simulink model "NCMS_AltMis_항공대"  (R2022a)
settings: Solver=FixedStepAuto  StartTime=0.0  StopTime=inf  FixedStep=SampleTime  RelTol=1e-3
InitFcn:
  | NCMS_AltMis_Init;
values from neighbouring files (symbols this model uses):
  Kdpr = 0.004    [NCMS_AltMis_Init_항공대.m]
  Kdrr = 0.004    [NCMS_AltMis_Init_항공대.m]
  Kdvz = 0.0254    [NCMS_AltMis_Init_항공대.m]
  Kdyr = 0.0298    [NCMS_AltMis_Init_항공대.m]
  Kipr = 0.1    [NCMS_AltMis_Init_항공대.m]
  Kirr = 0.1    [NCMS_AltMis_Init_항공대.m]
  Kivx = 0.0728/g    (= 0.00742099898063)    [NCMS_AltMis_Init_항공대.m]
  Kivy = 0.0728/g    (= 0.00742099898063)    [NCMS_AltMis_Init_항공대.m]
  Kivz = 0.6304    [NCMS_AltMis_Init_항공대.m]
  Kix = 0.02    [NCMS_AltMis_Init_항공대.m]
  Kiyaxis = 0.02    [NCMS_AltMis_Init_항공대.m]
  Kiyr = 0.7395    [NCMS_AltMis_Init_항공대.m]
  Kiz = 0.09    [NCMS_AltMis_Init_항공대.m]
  Kpp = 3.3894    [NCMS_AltMis_Init_항공대.m]
  Kppr = 0.1    [NCMS_AltMis_Init_항공대.m]
  Kpr = 3.3894    [NCMS_AltMis_Init_항공대.m]
  Kprr = 0.1    [NCMS_AltMis_Init_항공대.m]
  Kpvx = 2.1109/g    (= 0.215178389399)    [NCMS_AltMis_Init_항공대.m]
  Kpvy = 2.1109/g    (= 0.215178389399)    [NCMS_AltMis_Init_항공대.m]
  Kpvz = 0.3191    [NCMS_AltMis_Init_항공대.m]
  Kpx = 1    [NCMS_AltMis_Init_항공대.m]
  Kpy = 3.3894    [NCMS_AltMis_Init_항공대.m]
  Kpyaxis = 1    [NCMS_AltMis_Init_항공대.m]
  Kpyr = 0.3744    [NCMS_AltMis_Init_항공대.m]
  Kpz = 2.4    [NCMS_AltMis_Init_항공대.m]
  LAND_PRES_VEL = 0.2    [NCMS_AltMis_Init_항공대.m]
  MAX_CONTROL_ANGLE_PITCH = 30*pi/180    (= 0.523598775598)    [Init_FLIGHT_Hexacopter.m]    (also in NCMS_AltMis_Init_항공대.m = 0.349065850399)
  MAX_CONTROL_ANGLE_RATE_PITCH = 360*pi/180    (= 6.28318530718)    [Init_FLIGHT_Hexacopter.m]    (also in NCMS_AltMis_Init_항공대.m)
  MAX_CONTROL_ANGLE_RATE_ROLL = 360*pi/180    (= 6.28318530718)    [Init_FLIGHT_Hexacopter.m]    (also in NCMS_AltMis_Init_항공대.m)
  MAX_CONTROL_ANGLE_RATE_Y = 120*pi/180    (= 2.09439510239)    [Init_FLIGHT_Hexacopter.m]    (also in NCMS_AltMis_Init_항공대.m)
  MAX_CONTROL_ANGLE_ROLL = 30*pi/180    (= 0.523598775598)    [Init_FLIGHT_Hexacopter.m]    (also in NCMS_AltMis_Init_항공대.m = 0.349065850399)
  MAX_CONTROL_VELOCITY_XY = 1.5    [Init_FLIGHT_Hexacopter.m]    (also in NCMS_AltMis_Init_항공대.m)
  MAX_CONTROL_VELOCITY_Z = 1    [Init_FLIGHT_Hexacopter.m]    (also in NCMS_AltMis_Init_항공대.m)
  Npr = 50    [NCMS_AltMis_Init_항공대.m]
  Nrr = 50    [NCMS_AltMis_Init_항공대.m]
  Nvz = Npr    (= 50)    [NCMS_AltMis_Init_항공대.m]
  Nyr = 50    [NCMS_AltMis_Init_항공대.m]
  SampleTime = 1/250    (= 0.004)    [Init_FLIGHT_Hexacopter.m]    (also in NCMS_AltMis_Init_항공대.m = 0.01)
  THR_HOVER = 0.6085    [NCMS_AltMis_Init_항공대.m]
  THR_IDLE = 0.2    [NCMS_AltMis_Init_항공대.m]
undefined symbols (not defined in the file or in its folder): dev, Kdz, Main, Nz, pwm_output0
libraries: slpidlib x15, simulink x9, px4Sensorslib x3, px4uORBlib x3, uavalgslib x2, px4lib x1
(part 2 of 3)

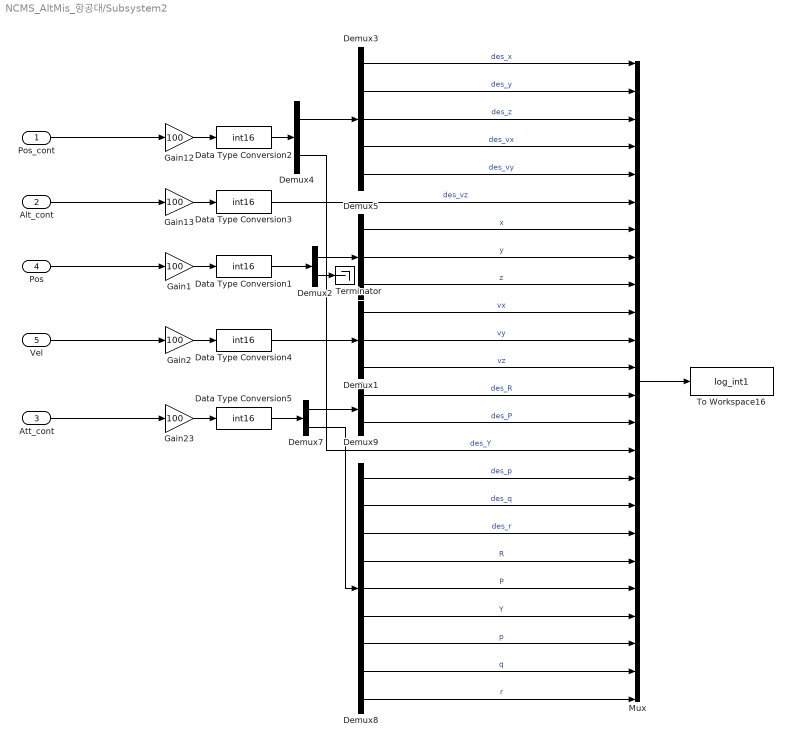
== system NCMS_AltMis_항공대/Subsystem2 ==
  Pos_cont : Inport
  Alt_cont : Inport  Port=2
  Att_cont : Inport  Port=3
  Pos : Inport  Port=4
  Vel : Inport  Port=5
  Data Type Conversion{1..5} (5 alike) : DataTypeConversion  OutDataTypeStr=int16  SaturateOnIntegerOverflow=off  RndMeth=Floor
  Demux1 : Demux  Outputs=3
  Demux2 : Demux  Outputs=[3 1]
  Demux3 : Demux  Outputs=5
  Demux4 : Demux  Outputs=[5 1]
  Demux5 : Demux  Outputs=3
  Demux7 : Demux  Outputs=[2 9]
  Demux8 : Demux  Outputs=9
  Demux9 : Demux  Outputs=2
  Gain{1..2,12..13,23} (5 alike) : Gain  Gain=100
  Mux : Mux  Inputs=24
  Terminator : Terminator
  To Workspace16 : ToWorkspace  VariableName=log_int1  SaveFormat=Structure  SampleTime=SampleTime
      settings: Save2DSignal=2-D array (concatenate along first dimension)
  wires:
  Att_cont/1 -> Gain23/1
  Data Type Conversion5/1 -> Demux7/1
  Data Type Conversion3/1 -> Mux/6  "des_vz"
  Data Type Conversion2/1 -> Demux4/1
  Demux2/2 -> Terminator/1
  Demux2/1 -> Demux5/1
  Data Type Conversion1/1 -> Demux2/1
  Data Type Conversion4/1 -> Demux1/1
  Gain2/1 -> Data Type Conversion4/1
  Demux1/3 -> Mux/12  "vz"
  Demux1/2 -> Mux/11  "vy"
  Demux1/1 -> Mux/10  "vx"
  Vel/1 -> Gain2/1
  Gain1/1 -> Data Type Conversion1/1
  Pos/1 -> Gain1/1
  Demux8/8 -> Mux/23  "q"
  Demux8/2 -> Mux/17  "des_q"
  Demux3/5 -> Mux/5  "des_vy"
  Demux8/9 -> Mux/24  "r"
  Gain23/1 -> Data Type Conversion5/1
  Demux5/3 -> Mux/9  "z"
  Demux5/2 -> Mux/8  "y"
  Mux/1 -> To Workspace16/1
  Demux3/1 -> Mux/1  "des_x"
  Pos_cont/1 -> Gain12/1
  Demux8/7 -> Mux/22  "p"
  Demux3/3 -> Mux/3  "des_z"
  Demux8/6 -> Mux/21  "Y"
  Demux4/1 -> Demux3/1
  Demux7/2 -> Demux8/1
  Demux7/1 -> Demux9/1
  Demux9/1 -> Mux/13  "des_R"
  Demux3/4 -> Mux/4  "des_vx"
  Alt_cont/1 -> Gain13/1
  Demux4/2 -> Mux/15  "des_Y"
  Demux8/3 -> Mux/18  "des_r"
  Demux3/2 -> Mux/2  "des_y"
  Demux8/1 -> Mux/16  "des_p"
  Gain12/1 -> Data Type Conversion2/1
  Demux8/5 -> Mux/20  "P"
  Demux5/1 -> Mux/7  "x"
  Demux8/4 -> Mux/19  "R"
  Gain13/1 -> Data Type Conversion3/1
  Demux9/2 -> Mux/14  "des_P"

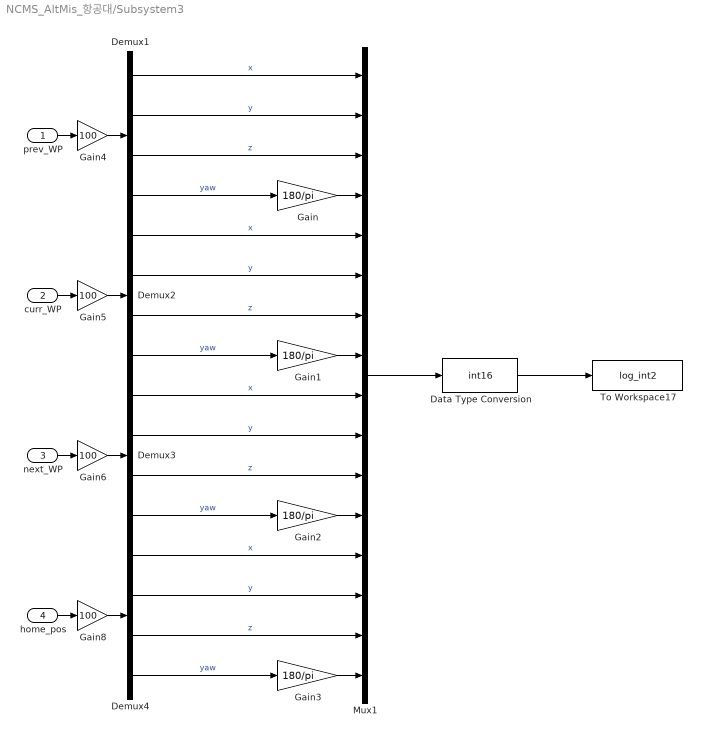
== system NCMS_AltMis_항공대/Subsystem3 ==
  prev_WP : Inport
  curr_WP : Inport  Port=2
  next_WP : Inport  Port=3
  home_pos : Inport  Port=4
  Data Type Conversion : DataTypeConversion  OutDataTypeStr=int16  SaturateOnIntegerOverflow=off  RndMeth=Floor
  Demux{1..4} (4 alike) : Demux
  Gain{,1..3} (4 alike) : Gain  Gain=180/pi
  Gain{4..6,8} (4 alike) : Gain  Gain=100
  Mux1 : Mux  Inputs=16
  To Workspace17 : ToWorkspace  VariableName=log_int2  SaveFormat=Structure  SampleTime=SampleTime
      settings: Save2DSignal=2-D array (concatenate along first dimension)
  wires:
  Mux1/1 -> Data Type Conversion/1
  Demux1/4 -> Gain/1  "yaw"
  prev_WP/1 -> Gain4/1
  Demux1/1 -> Mux1/1  "x"
  Demux1/2 -> Mux1/2  "y"
  Demux1/3 -> Mux1/3  "z"
  Demux2/4 -> Gain1/1  "yaw"
  Demux2/3 -> Mux1/7  "z"
  Demux2/1 -> Mux1/5  "x"
  Demux2/2 -> Mux1/6  "y"
  Demux3/4 -> Gain2/1  "yaw"
  Demux3/3 -> Mux1/11  "z"
  Demux3/1 -> Mux1/9  "x"
  Demux3/2 -> Mux1/10  "y"
  Demux4/4 -> Gain3/1  "yaw"
  Demux4/3 -> Mux1/15  "z"
  Demux4/1 -> Mux1/13  "x"
  Demux4/2 -> Mux1/14  "y"
  curr_WP/1 -> Gain5/1
  next_WP/1 -> Gain6/1
  home_pos/1 -> Gain8/1
  Gain4/1 -> Demux1/1
  Gain5/1 -> Demux2/1
  Gain6/1 -> Demux3/1
  Gain8/1 -> Demux4/1
  Gain/1 -> Mux1/4
  Gain1/1 -> Mux1/8
  Gain2/1 -> Mux1/12
  Gain3/1 -> Mux1/16
  Data Type Conversion/1 -> To Workspace17/1

== system NCMS_AltMis_항공대/Vz Controller ==
  des_vz : Inport
  vz : Inport  Port=2
  All_reset : Inport  Port=3
  Gain : Gain  Gain=-1
  Hovering Thrust : Constant  Value=THR_HOVER  OutDataTypeStr=single  SampleTime=SampleTime
  PID Controller4 : slpidlib/PID Controller  Controller=PID  Form=Parallel  TimeDomain=Discrete-time  UseExternalTs=off  SampleTime=SampleTime  IntegratorMethod=Forward Euler  FilterMethod=Forward Euler  ControllerParametersSource=internal  P=Kpvz  I=Kivz  UseKiTs=off  D=Kdvz  N=Nvz  UseFilter=on  TunerSelectOption=Transfer Function Based (PID Tuner App)  InitialConditionSource=internal  InitialConditionForIntegrator=0  InitialConditionForFilter=0  DifferentiatorICPrevScaledInput=0  ExternalReset=either  TrackingMode=off  Kt=1  LimitOutput=on  SatLimitsSource=internal  UpperSaturationLimit=1  LowerSaturationLimit=-1  LinearizeAsGain=on  AntiWindupMode=clamping  Kb=1  POutMin=[]  POutMax=[]  IOutMin=[]  IOutMax=[]  DOutMin=[]  DOutMax=[]  NOutMin=[]  NOutMax=[]  SumOutMin=[]  SumOutMax=[]  SaturationOutMin=[]  SaturationOutMax=[]  PParamMin=[]  PParamMax=[]  IParamMin=[]  IParamMax=[]  DParamMin=[]  DParamMax=[]  NParamMin=[]  NParamMax=[]  KbParamMin=[]  KbParamMax=[]  KtParamMin=[]  KtParamMax=[]  KbOutMin=[]  KbOutMax=[]  KtOutMin=[]  KtOutMax=[]  IntegratorOutMin=[]  IntegratorOutMax=[]  FilterOutMin=[]  FilterOutMax=[]  SumI1OutMin=[]  SumI1OutMax=[]  SumI2OutMin=[]  SumI2OutMax=[]  SumI3OutMin=[]  SumI3OutMax=[]  SumI4OutMin=[]  SumI4OutMax=[]  SumDOutMin=[]  SumDOutMax=[]  DifferentiatorOutMin=[]  DifferentiatorOutMax=[]  FilterDiffOutCoefMin=[]  FilterDiffOutCoefMax=[]  ReciprocalOutMin=[]  ReciprocalOutMax=[]  SumDenOutMin=[]  SumDenOutMax=[]  SumNumOutMin=[]  SumNumOutMax=[]  DivideOutMin=[]  DivideOutMax=[]  UdiffTsProdOutMin=[]  UdiffTsProdOutMax=[]  NTsProdOutMin=[]  NTsProdOutMax=[]  UintegralTsProdOutMin=[]  UintegralTsProdOutMax=[]  UngainTsProdOutMin=[]  UngainTsProdOutMax=[]  IntegratorContinuousStateAttributes=''  IntegratorStateMustResolveToSignalObject=off  IntegratorRTWStateStorageClass=Auto  FilterContinuousStateAttributes=''  FilterStateMustResolveToSignalObject=off  FilterRTWStateStorageClass=Auto  ParallelPVariant=InternalParameters  IdealPVariant=Disabled  IVariant=InternalParameters  DVariant=InternalParameters  IntegratorVariant=Discrete  SatVariant=Enabled  AWVariant=DiscClampingParallel  PCopyVariant=Disabled  TRVariant=Disabled  FdbkBlocksVariant=Forward  IdealPFdbkVariant=Disabled  SatFdbkVariant=Disabled  DerivativeFilterVariant=ForwardEulerFilter  NVariant=InternalParameters  NCopyVariant=Disabled  FilterICVariant=InternalICsFilter  IntegratorICVariant=InternalICs  ExternalResetVariant=ExternalReset  TRSumVariant=Passthrough  SumFdbkVariant=Disabled  SumVariant=Sum_PID  TsampFilterVariant=InternalTs  TsampNgainVariant=Passthrough  TsampIntegralVariant=Passthrough  ExternalSaturationOutDataTypeStr=Inherit: Same as second input  aMode=0
  Saturation1 : Saturate  UpperLimit=1  LowerLimit=0  OutDataTypeStr=single
  Sum3 : Sum  Inputs=|+-
  Sum6 : Sum  Inputs=|++  OutDataTypeStr=single
  f : Outport  OutDataTypeStr=single
  log_alt : Outport  Port=2  OutDataTypeStr=single
  wires:
  Saturation1/1 -> f/1
  All_reset/1 -> PID Controller4/2
  vz/1 -> Sum3/2
  des_vz/1 -> [des_vz], Sum3/1
  Sum3/1 -> Gain/1
  Gain/1 -> PID Controller4/1
  PID Controller4/1 -> Sum6/1
  Sum6/1 -> Saturation1/1
  Hovering Thrust/1 -> Sum6/2
  [des_vz] -> log_alt/1

== system NCMS_AltMis_항공대/Guidance/IDLE or Hovering ==
  Current Position : Inport
  Action Port : ActionPort  InitializeStates=reset  ActionPortLabel=else
  Maintain Current Yaw during IDLE : Subsystem
  Mux : Mux  Inputs=2
  Reshape1 : Reshape  OutputDimensionality=Row vector (2-D)
  Selector : Selector  InputPortWidth=4  IndexOptions=Index vector (dialog)  Indices=[4]  OutputSizes=1
  Selector1 : Selector  InputPortWidth=4  IndexOptions=Index vector (dialog)  Indices=[1 2 3]  OutputSizes=1
  x_y_z_yaw : Outport
  wires:
  Maintain Current Yaw during IDLE/1(yaw_Out) -> Mux/2
  Current Position/1 -> Selector/1, Selector1/1
  Selector/1 -> Maintain Current Yaw during IDLE/1(yaw_In)
  Selector1/1 -> Mux/1
  Mux/1 -> Reshape1/1
  Reshape1/1 -> x_y_z_yaw/1

== system NCMS_AltMis_항공대/Guidance/Land ==
  Current Position : Inport
  Current WP : Inport  Port=2
  Previous WP : Inport  Port=3
  type : Inport  Port=4
  Action Port : ActionPort  InitializeStates=reset  ActionPortLabel=elseif(u1 ==4)
  Delay : Delay  DelayLength=1
  Ensure Smooth descend during Land : Subsystem
  IsNaN : RelationalOperator  Operator=isNaN  OutDataTypeStr=boolean  RndMeth=Simplest  InputSameDT=off
  Maintain Current Yaw during Land : Subsystem
  Mux : Mux  Inputs=3
  OR : Logic  Operator=OR  Inputs=1  IconShape=distinctive  AllPortsSameDT=off  OutDataTypeStr=boolean
  Reshape : Reshape  OutputDimensionality=Row vector (2-D)
  Reshape1 : Reshape  OutputDimensionality=Row vector (2-D)
  Selector : Selector  InputPortWidth=4  IndexOptions=Index vector (dialog)  Indices=[4]  OutputSizes=1
  Selector1 : Selector  InputPortWidth=4  IndexOptions=Index vector (dialog)  Indices=[1 2]  OutputSizes=1
  Selector2 : Selector  InputPortWidth=4  IndexOptions=Index vector (dialog)  Indices=[1 2]  OutputSizes=1
  Switch : Switch  Criteria=u2 > Threshold  SaturateOnIntegerOverflow=off  InputSameDT=off
  x_y_z_yaw : Outport
  wires:
  Delay/1 -> Switch/1
  Reshape1/1 -> Delay/1
  OR/1 -> Switch/2
  Mux/1 -> Reshape/1
  Selector1/1 -> Switch/3, IsNaN/1
  Reshape/1 -> x_y_z_yaw/1
  Current Position/1 -> Ensure Smooth descend during Land/3(Current Position), Selector/1, Selector2/1
  IsNaN/1 -> OR/1
  Selector2/1 -> Reshape1/1
  Current WP/1 -> Ensure Smooth descend during Land/2(Current WP), Selector1/1
  Switch/1 -> Mux/1
  Previous WP/1 -> Ensure Smooth descend during Land/1(Previous WP)
  Maintain Current Yaw during Land/1(yaw_Out) -> Mux/3
  Selector/1 -> Maintain Current Yaw during Land/1(yaw_In)
  type/1 -> Ensure Smooth descend during Land/4(type)
  Ensure Smooth descend during Land/1(z) -> Mux/2

== system NCMS_AltMis_항공대/Guidance/Take-off ==
  Current Position : Inport
  Current WP : Inport  Port=2
  Action Port : ActionPort  InitializeStates=reset  ActionPortLabel=if((u1 ==3))
  Demux : Demux
  Demux1 : Demux
  Ensure smooth ascend during Takeoff : Subsystem
  Maintain Current Yaw during TakeOff : Subsystem
  Mux : Mux
  Reshape : Reshape  OutputDimensionality=Row vector (2-D)
  Terminator{,1..3} (4 alike) : Terminator
  x_y_z_yaw : Outport
  wires:
  Current Position/1 -> Demux/1
  Mux/1 -> Reshape/1
  Current WP/1 -> Demux1/1
  Demux1/3 -> Ensure smooth ascend during Takeoff/1(" ")
  Demux/3 -> Terminator3/1
  Demux/1 -> Terminator1/1
  Demux/2 -> Terminator2/1
  Demux1/1 -> Mux/1
  Demux1/2 -> Mux/2
  Reshape/1 -> x_y_z_yaw/1
  Demux/4 -> Maintain Current Yaw during TakeOff/1(yaw_In)
  Maintain Current Yaw during TakeOff/1(yaw_Out) -> Mux/4
  Ensure smooth ascend during Takeoff/1(Out1) -> Mux/3
  Demux1/4 -> Terminator/1

== system NCMS_AltMis_항공대/Guidance/Waypoint ==
  Current Position : Inport
  Previous WP : Inport  Port=2
  Current WP : Inport  Port=3
  Next WP : Inport  Port=4
  Waypoint Type : Inport  Port=5
  Action Port : ActionPort  InitializeStates=reset  ActionPortLabel=elseif( u1==0)
  IsNaN : RelationalOperator  Operator=isNaN  OutDataTypeStr=boolean  RndMeth=Simplest  InputSameDT=off
  Look-ahead Calculation : Subsystem
  Output signal conditioning : Subsystem
  Selector2 : Selector  InputPortWidth=4  IndexOptions=Index vector (dialog)  Indices=4  OutputSizes=1
  Switch : Switch  Criteria=u2 ~= 0  SaturateOnIntegerOverflow=off  InputSameDT=off
  Switch1 : Switch  Criteria=u2 ~= 0  SaturateOnIntegerOverflow=off  InputSameDT=off
  Terminator1 : Terminator
  Terminator2 : Terminator
  UAV Waypoint Follower : uavalgslib/Waypoint Follower  UAVType=multirotor  StartFrom=first  TransitionRadiusSource=internal  TransitionRadius=Transition_radius  MinLookaheadDistance=1  YawInput=on  ShowCrossTrackErrorOutput=off  ShowStatusOutput=off  SimulateUsing=Code generation
      settings: SourceProductBaseCode=UV
  UAV Waypoint Follower1 : uavalgslib/Waypoint Follower  UAVType=multirotor  StartFrom=first  TransitionRadiusSource=internal  TransitionRadius=Transition_radius  MinLookaheadDistance=1  YawInput=off  ShowCrossTrackErrorOutput=off  ShowStatusOutput=off  SimulateUsing=Code generation
      settings: SourceProductBaseCode=UV
  for fixedwing : Terminator
  for fixedwing1 : Terminator
  x_y_z_yaw : Outport
  wires:
  Look-ahead Calculation/3(LookAhead) -> UAV Waypoint Follower1/3, UAV Waypoint Follower/3
  Current WP/1 -> Selector2/1, Look-ahead Calculation/3(current)
  Previous WP/1 -> Look-ahead Calculation/2(previous)
  Look-ahead Calculation/2(WP_pose) -> UAV Waypoint Follower/2
  UAV Waypoint Follower/2 -> for fixedwing/1
  Look-ahead Calculation/1(Pose) -> UAV Waypoint Follower/1, UAV Waypoint Follower1/1
  Output signal conditioning/1(xyzYaw) -> x_y_z_yaw/1
  Waypoint Type/1 -> Output signal conditioning/4(Waypoint Type)
  UAV Waypoint Follower/4 -> Terminator1/1
  Current Position/1 -> Output signal conditioning/1(Current Position), Look-ahead Calculation/1(Estimated Pos)
  Next WP/1 -> Look-ahead Calculation/4(next)
  Look-ahead Calculation/4(WP_pos) -> UAV Waypoint Follower1/2
  UAV Waypoint Follower1/2 -> for fixedwing1/1
  UAV Waypoint Follower1/4 -> Terminator2/1
  IsNaN/1 -> Switch1/2, Switch/2
  Selector2/1 -> IsNaN/1
  Switch/1 -> Output signal conditioning/2(LookAhead Point)
  Switch1/1 -> Output signal conditioning/3(Desired Yaw)
  UAV Waypoint Follower1/1 -> Switch/1
  UAV Waypoint Follower1/3 -> Switch1/1
  UAV Waypoint Follower/1 -> Switch/3
  UAV Waypoint Follower/3 -> Switch1/3

== system NCMS_AltMis_항공대/Mixer/If Action Subsystem ==
  Roll : Inport
  Pitch : Inport  Port=2
  Yaw : Inport  Port=3
  Thrust : Inport  Port=4
  Action Port : ActionPort  InitializeStates=reset  ActionPortLabel=if((u1 == 1)&(u2 == 0))
  Mux : Mux
  pwm_out2 : MATLAB Function  SystemSampleTime=0.004
  Out1 : Outport
  wires:
  pwm_out2/3(M3) -> Mux/3
  Pitch/1 -> pwm_out2/2(Pitch)
  Yaw/1 -> pwm_out2/3(Yaw)
  pwm_out2/2(M2) -> Mux/2
  Thrust/1 -> pwm_out2/4(Thrust)
  Roll/1 -> pwm_out2/1(Roll)
  pwm_out2/4(M4) -> Mux/4
  pwm_out2/1(M1) -> Mux/1
  Mux/1 -> Out1/1

== system NCMS_AltMis_항공대/Mixer/If Action Subsystem1 ==
  Roll : Inport
  Pitch : Inport  Port=2
  Yaw : Inport  Port=3
  Thrust : Inport  Port=4
  Action Port : ActionPort  InitializeStates=reset  ActionPortLabel=elseif((u1 ~= 1)&(u3 == 0))
  Mux : Mux
  pwm_out2 : MATLAB Function  SystemSampleTime=0.004
  Out1 : Outport
  wires:
  pwm_out2/3(M3) -> Mux/3
  Pitch/1 -> pwm_out2/2(Pitch)
  Yaw/1 -> pwm_out2/3(Yaw)
  pwm_out2/2(M2) -> Mux/2
  Thrust/1 -> pwm_out2/4(Thrust)
  Roll/1 -> pwm_out2/1(Roll)
  pwm_out2/4(M4) -> Mux/4
  pwm_out2/1(M1) -> Mux/1
  Mux/1 -> Out1/1

== system NCMS_AltMis_항공대/Mixer/If Action Subsystem2 ==
  Roll : Inport
  Pitch : Inport  Port=2
  Yaw : Inport  Port=3
  Thrust : Inport  Port=4
  Action Port : ActionPort  InitializeStates=reset  ActionPortLabel=else
  Mux : Mux
  pwm_out2 : MATLAB Function  SystemSampleTime=0.004
  Out1 : Outport
  wires:
  pwm_out2/3(M3) -> Mux/3
  Pitch/1 -> pwm_out2/2(Pitch)
  Yaw/1 -> pwm_out2/3(Yaw)
  pwm_out2/2(M2) -> Mux/2
  Thrust/1 -> pwm_out2/4(Thrust)
  Roll/1 -> pwm_out2/1(Roll)
  pwm_out2/4(M4) -> Mux/4
  pwm_out2/1(M1) -> Mux/1
  Mux/1 -> Out1/1

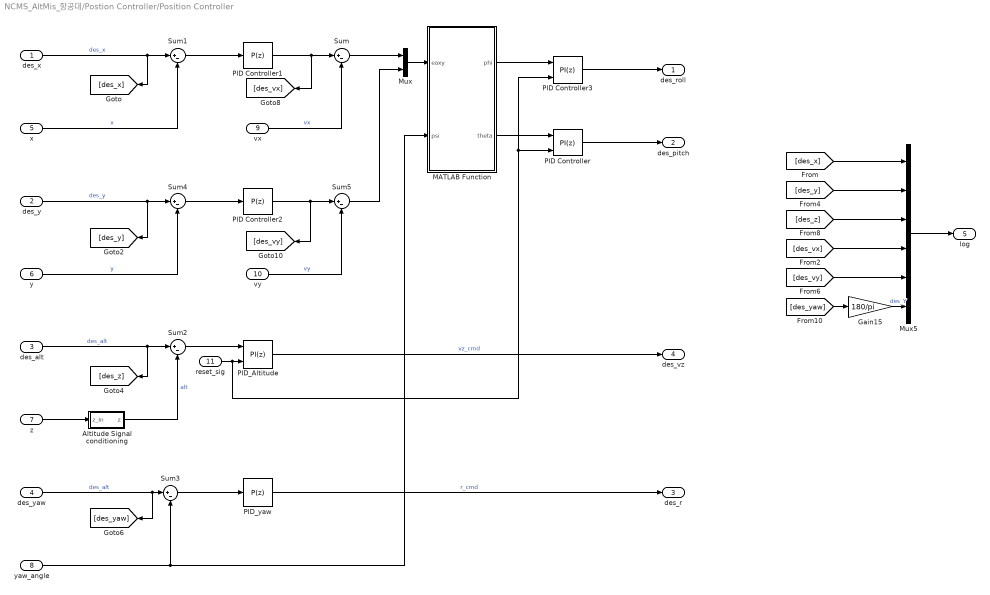
== system NCMS_AltMis_항공대/Postion Controller/Position Controller ==
  des_x : Inport
  des_y : Inport  Port=2
  des_alt : Inport  Port=3
  des_yaw : Inport  Port=4
  x : Inport  Port=5
  y : Inport  Port=6
  z : Inport  Port=7
  yaw_angle : Inport  Port=8
  vx : Inport  Port=9
  vy : Inport  Port=10
  reset_sig : Inport  Port=11
  Altitude Signal conditioning : Subsystem
  Gain15 : Gain  Gain=180/pi
  MATLAB Function : MATLAB Function  TreatAsAtomicUnit=on
  Mux : Mux  Inputs=2
  Mux5 : Mux  Inputs=6
  PID Controller : slpidlib/PID Controller  Controller=PI  Form=Parallel  TimeDomain=Discrete-time  UseExternalTs=off  SampleTime=SampleTime  IntegratorMethod=Forward Euler  FilterMethod=Forward Euler  ControllerParametersSource=internal  P=Kpvx  I=Kivx  UseKiTs=off  D=0  N=20  UseFilter=on  TunerSelectOption=Transfer Function Based (PID Tuner App)  InitialConditionSource=internal  InitialConditionForIntegrator=0  InitialConditionForFilter=0  DifferentiatorICPrevScaledInput=0  ExternalReset=either  TrackingMode=off  Kt=1  LimitOutput=on  SatLimitsSource=internal  UpperSaturationLimit=MAX_CONTROL_ANGLE_PITCH  LowerSaturationLimit=-MAX_CONTROL_ANGLE_PITCH  LinearizeAsGain=on  AntiWindupMode=clamping  Kb=1  POutMin=[]  POutMax=[]  IOutMin=[]  IOutMax=[]  DOutMin=[]  DOutMax=[]  NOutMin=[]  NOutMax=[]  SumOutMin=[]  SumOutMax=[]  SaturationOutMin=[]  SaturationOutMax=[]  PParamMin=[]  PParamMax=[]  IParamMin=[]  IParamMax=[]  DParamMin=[]  DParamMax=[]  NParamMin=[]  NParamMax=[]  KbParamMin=[]  KbParamMax=[]  KtParamMin=[]  KtParamMax=[]  KbOutMin=[]  KbOutMax=[]  KtOutMin=[]  KtOutMax=[]  IntegratorOutMin=[]  IntegratorOutMax=[]  FilterOutMin=[]  FilterOutMax=[]  SumI1OutMin=[]  SumI1OutMax=[]  SumI2OutMin=[]  SumI2OutMax=[]  SumI3OutMin=[]  SumI3OutMax=[]  SumI4OutMin=[]  SumI4OutMax=[]  SumDOutMin=[]  SumDOutMax=[]  DifferentiatorOutMin=[]  DifferentiatorOutMax=[]  FilterDiffOutCoefMin=[]  FilterDiffOutCoefMax=[]  ReciprocalOutMin=[]  ReciprocalOutMax=[]  SumDenOutMin=[]  SumDenOutMax=[]  SumNumOutMin=[]  SumNumOutMax=[]  DivideOutMin=[]  DivideOutMax=[]  UdiffTsProdOutMin=[]  UdiffTsProdOutMax=[]  NTsProdOutMin=[]  NTsProdOutMax=[]  UintegralTsProdOutMin=[]  UintegralTsProdOutMax=[]  UngainTsProdOutMin=[]  UngainTsProdOutMax=[]  IntegratorContinuousStateAttributes=''  IntegratorStateMustResolveToSignalObject=off  IntegratorRTWStateStorageClass=Auto  FilterContinuousStateAttributes=''  FilterStateMustResolveToSignalObject=off  FilterRTWStateStorageClass=Auto  ParallelPVariant=InternalParameters  IdealPVariant=Disabled  IVariant=InternalParameters  DVariant=Disabled  IntegratorVariant=Discrete  SatVariant=Enabled  AWVariant=DiscClampingParallel  PCopyVariant=Disabled  TRVariant=Disabled  FdbkBlocksVariant=Forward  IdealPFdbkVariant=Disabled  SatFdbkVariant=Disabled  DerivativeFilterVariant=Disabled  NVariant=Disabled  NCopyVariant=Disabled_SignalSpec  FilterICVariant=Disabled  IntegratorICVariant=InternalICs  ExternalResetVariant=ExternalReset  TRSumVariant=Passthrough  SumFdbkVariant=Disabled  SumVariant=Sum_PI  TsampFilterVariant=InternalTs  TsampNgainVariant=Passthrough  TsampIntegralVariant=Passthrough  ExternalSaturationOutDataTypeStr=Inherit: Same as second input  aMode=0
  PID Controller1 : slpidlib/PID Controller  Controller=P  Form=Parallel  TimeDomain=Discrete-time  UseExternalTs=off  SampleTime=SampleTime  IntegratorMethod=Forward Euler  FilterMethod=Forward Euler  ControllerParametersSource=internal  P=Kpx  I=Kix  UseKiTs=off  D=0  N=20  UseFilter=on  TunerSelectOption=Transfer Function Based (PID Tuner App)  InitialConditionSource=internal  InitialConditionForIntegrator=0  InitialConditionForFilter=0  DifferentiatorICPrevScaledInput=0  ExternalReset=either  TrackingMode=off  Kt=1  LimitOutput=on  SatLimitsSource=internal  UpperSaturationLimit=MAX_CONTROL_VELOCITY_XY  LowerSaturationLimit=-MAX_CONTROL_VELOCITY_XY  LinearizeAsGain=on  AntiWindupMode=clamping  Kb=1  POutMin=[]  POutMax=[]  IOutMin=[]  IOutMax=[]  DOutMin=[]  DOutMax=[]  NOutMin=[]  NOutMax=[]  SumOutMin=[]  SumOutMax=[]  SaturationOutMin=[]  SaturationOutMax=[]  PParamMin=[]  PParamMax=[]  IParamMin=[]  IParamMax=[]  DParamMin=[]  DParamMax=[]  NParamMin=[]  NParamMax=[]  KbParamMin=[]  KbParamMax=[]  KtParamMin=[]  KtParamMax=[]  KbOutMin=[]  KbOutMax=[]  KtOutMin=[]  KtOutMax=[]  IntegratorOutMin=[]  IntegratorOutMax=[]  FilterOutMin=[]  FilterOutMax=[]  SumI1OutMin=[]  SumI1OutMax=[]  SumI2OutMin=[]  SumI2OutMax=[]  SumI3OutMin=[]  SumI3OutMax=[]  SumI4OutMin=[]  SumI4OutMax=[]  SumDOutMin=[]  SumDOutMax=[]  DifferentiatorOutMin=[]  DifferentiatorOutMax=[]  FilterDiffOutCoefMin=[]  FilterDiffOutCoefMax=[]  ReciprocalOutMin=[]  ReciprocalOutMax=[]  SumDenOutMin=[]  SumDenOutMax=[]  SumNumOutMin=[]  SumNumOutMax=[]  DivideOutMin=[]  DivideOutMax=[]  UdiffTsProdOutMin=[]  UdiffTsProdOutMax=[]  NTsProdOutMin=[]  NTsProdOutMax=[]  UintegralTsProdOutMin=[]  UintegralTsProdOutMax=[]  UngainTsProdOutMin=[]  UngainTsProdOutMax=[]  IntegratorContinuousStateAttributes=''  IntegratorStateMustResolveToSignalObject=off  IntegratorRTWStateStorageClass=Auto  FilterContinuousStateAttributes=''  FilterStateMustResolveToSignalObject=off  FilterRTWStateStorageClass=Auto  ParallelPVariant=InternalParameters  IdealPVariant=Disabled  IVariant=Disabled  DVariant=Disabled  IntegratorVariant=Disabled  SatVariant=Enabled  AWVariant=Disabled  PCopyVariant=Disabled  TRVariant=Disabled  FdbkBlocksVariant=Forward  IdealPFdbkVariant=Disabled  SatFdbkVariant=Disabled  DerivativeFilterVariant=Disabled  NVariant=Disabled  NCopyVariant=Disabled_SignalSpec  FilterICVariant=Disabled  IntegratorICVariant=Disabled  ExternalResetVariant=Disabled  TRSumVariant=Passthrough  SumFdbkVariant=Disabled  SumVariant=Passthrough_P  TsampFilterVariant=InternalTs  TsampNgainVariant=Passthrough  TsampIntegralVariant=Disabled_SignalSpec  ExternalSaturationOutDataTypeStr=Inherit: Same as second input  aMode=0
  PID Controller2 : slpidlib/PID Controller  Controller=P  Form=Parallel  TimeDomain=Discrete-time  UseExternalTs=off  SampleTime=SampleTime  IntegratorMethod=Forward Euler  FilterMethod=Forward Euler  ControllerParametersSource=internal  P=Kpyaxis  I=Kiyaxis  UseKiTs=off  D=0  N=20  UseFilter=on  TunerSelectOption=Transfer Function Based (PID Tuner App)  InitialConditionSource=internal  InitialConditionForIntegrator=0  InitialConditionForFilter=0  DifferentiatorICPrevScaledInput=0  ExternalReset=either  TrackingMode=off  Kt=1  LimitOutput=on  SatLimitsSource=internal  UpperSaturationLimit=MAX_CONTROL_VELOCITY_XY  LowerSaturationLimit=-MAX_CONTROL_VELOCITY_XY  LinearizeAsGain=on  AntiWindupMode=clamping  Kb=1  POutMin=[]  POutMax=[]  IOutMin=[]  IOutMax=[]  DOutMin=[]  DOutMax=[]  NOutMin=[]  NOutMax=[]  SumOutMin=[]  SumOutMax=[]  SaturationOutMin=[]  SaturationOutMax=[]  PParamMin=[]  PParamMax=[]  IParamMin=[]  IParamMax=[]  DParamMin=[]  DParamMax=[]  NParamMin=[]  NParamMax=[]  KbParamMin=[]  KbParamMax=[]  KtParamMin=[]  KtParamMax=[]  KbOutMin=[]  KbOutMax=[]  KtOutMin=[]  KtOutMax=[]  IntegratorOutMin=[]  IntegratorOutMax=[]  FilterOutMin=[]  FilterOutMax=[]  SumI1OutMin=[]  SumI1OutMax=[]  SumI2OutMin=[]  SumI2OutMax=[]  SumI3OutMin=[]  SumI3OutMax=[]  SumI4OutMin=[]  SumI4OutMax=[]  SumDOutMin=[]  SumDOutMax=[]  DifferentiatorOutMin=[]  DifferentiatorOutMax=[]  FilterDiffOutCoefMin=[]  FilterDiffOutCoefMax=[]  ReciprocalOutMin=[]  ReciprocalOutMax=[]  SumDenOutMin=[]  SumDenOutMax=[]  SumNumOutMin=[]  SumNumOutMax=[]  DivideOutMin=[]  DivideOutMax=[]  UdiffTsProdOutMin=[]  UdiffTsProdOutMax=[]  NTsProdOutMin=[]  NTsProdOutMax=[]  UintegralTsProdOutMin=[]  UintegralTsProdOutMax=[]  UngainTsProdOutMin=[]  UngainTsProdOutMax=[]  IntegratorContinuousStateAttributes=''  IntegratorStateMustResolveToSignalObject=off  IntegratorRTWStateStorageClass=Auto  FilterContinuousStateAttributes=''  FilterStateMustResolveToSignalObject=off  FilterRTWStateStorageClass=Auto  ParallelPVariant=InternalParameters  IdealPVariant=Disabled  IVariant=Disabled  DVariant=Disabled  IntegratorVariant=Disabled  SatVariant=Enabled  AWVariant=Disabled  PCopyVariant=Disabled  TRVariant=Disabled  FdbkBlocksVariant=Forward  IdealPFdbkVariant=Disabled  SatFdbkVariant=Disabled  DerivativeFilterVariant=Disabled  NVariant=Disabled  NCopyVariant=Disabled_SignalSpec  FilterICVariant=Disabled  IntegratorICVariant=Disabled  ExternalResetVariant=Disabled  TRSumVariant=Passthrough  SumFdbkVariant=Disabled  SumVariant=Passthrough_P  TsampFilterVariant=InternalTs  TsampNgainVariant=Passthrough  TsampIntegralVariant=Disabled_SignalSpec  ExternalSaturationOutDataTypeStr=Inherit: Same as second input  aMode=0
  PID Controller3 : slpidlib/PID Controller  Controller=PI  Form=Parallel  TimeDomain=Discrete-time  UseExternalTs=off  SampleTime=SampleTime  IntegratorMethod=Forward Euler  FilterMethod=Forward Euler  ControllerParametersSource=internal  P=Kpvy  I=Kivy  UseKiTs=off  D=0  N=20  UseFilter=on  TunerSelectOption=Transfer Function Based (PID Tuner App)  InitialConditionSource=internal  InitialConditionForIntegrator=0  InitialConditionForFilter=0  DifferentiatorICPrevScaledInput=0  ExternalReset=either  TrackingMode=off  Kt=1  LimitOutput=on  SatLimitsSource=internal  UpperSaturationLimit=MAX_CONTROL_ANGLE_ROLL  LowerSaturationLimit=-MAX_CONTROL_ANGLE_ROLL  LinearizeAsGain=on  AntiWindupMode=clamping  Kb=1  POutMin=[]  POutMax=[]  IOutMin=[]  IOutMax=[]  DOutMin=[]  DOutMax=[]  NOutMin=[]  NOutMax=[]  SumOutMin=[]  SumOutMax=[]  SaturationOutMin=[]  SaturationOutMax=[]  PParamMin=[]  PParamMax=[]  IParamMin=[]  IParamMax=[]  DParamMin=[]  DParamMax=[]  NParamMin=[]  NParamMax=[]  KbParamMin=[]  KbParamMax=[]  KtParamMin=[]  KtParamMax=[]  KbOutMin=[]  KbOutMax=[]  KtOutMin=[]  KtOutMax=[]  IntegratorOutMin=[]  IntegratorOutMax=[]  FilterOutMin=[]  FilterOutMax=[]  SumI1OutMin=[]  SumI1OutMax=[]  SumI2OutMin=[]  SumI2OutMax=[]  SumI3OutMin=[]  SumI3OutMax=[]  SumI4OutMin=[]  SumI4OutMax=[]  SumDOutMin=[]  SumDOutMax=[]  DifferentiatorOutMin=[]  DifferentiatorOutMax=[]  FilterDiffOutCoefMin=[]  FilterDiffOutCoefMax=[]  ReciprocalOutMin=[]  ReciprocalOutMax=[]  SumDenOutMin=[]  SumDenOutMax=[]  SumNumOutMin=[]  SumNumOutMax=[]  DivideOutMin=[]  DivideOutMax=[]  UdiffTsProdOutMin=[]  UdiffTsProdOutMax=[]  NTsProdOutMin=[]  NTsProdOutMax=[]  UintegralTsProdOutMin=[]  UintegralTsProdOutMax=[]  UngainTsProdOutMin=[]  UngainTsProdOutMax=[]  IntegratorContinuousStateAttributes=''  IntegratorStateMustResolveToSignalObject=off  IntegratorRTWStateStorageClass=Auto  FilterContinuousStateAttributes=''  FilterStateMustResolveToSignalObject=off  FilterRTWStateStorageClass=Auto  ParallelPVariant=InternalParameters  IdealPVariant=Disabled  IVariant=InternalParameters  DVariant=Disabled  IntegratorVariant=Discrete  SatVariant=Enabled  AWVariant=DiscClampingParallel  PCopyVariant=Disabled  TRVariant=Disabled  FdbkBlocksVariant=Forward  IdealPFdbkVariant=Disabled  SatFdbkVariant=Disabled  DerivativeFilterVariant=Disabled  NVariant=Disabled  NCopyVariant=Disabled_SignalSpec  FilterICVariant=Disabled  IntegratorICVariant=InternalICs  ExternalResetVariant=ExternalReset  TRSumVariant=Passthrough  SumFdbkVariant=Disabled  SumVariant=Sum_PI  TsampFilterVariant=InternalTs  TsampNgainVariant=Passthrough  TsampIntegralVariant=Passthrough  ExternalSaturationOutDataTypeStr=Inherit: Same as second input  aMode=0
  PID_Altitude : slpidlib/PID Controller  Controller=PI  Form=Parallel  TimeDomain=Discrete-time  UseExternalTs=off  SampleTime=SampleTime  IntegratorMethod=Backward Euler  FilterMethod=Forward Euler  ControllerParametersSource=internal  P=Kpz  I=Kiz  UseKiTs=off  D=Kdz  N=Nz  UseFilter=on  TunerSelectOption=Transfer Function Based (PID Tuner App)  InitialConditionSource=internal  InitialConditionForIntegrator=0  InitialConditionForFilter=0  DifferentiatorICPrevScaledInput=0  ExternalReset=either  TrackingMode=off  Kt=1  LimitOutput=on  SatLimitsSource=internal  UpperSaturationLimit=MAX_CONTROL_VELOCITY_Z  LowerSaturationLimit=-MAX_CONTROL_VELOCITY_Z  LinearizeAsGain=off  AntiWindupMode=clamping  Kb=1  POutMin=[]  POutMax=[]  IOutMin=[]  IOutMax=[]  DOutMin=[]  DOutMax=[]  NOutMin=[]  NOutMax=[]  SumOutMin=[]  SumOutMax=[]  SaturationOutMin=[]  SaturationOutMax=[]  PParamMin=[]  PParamMax=[]  IParamMin=[]  IParamMax=[]  DParamMin=[]  DParamMax=[]  NParamMin=[]  NParamMax=[]  KbParamMin=[]  KbParamMax=[]  KtParamMin=[]  KtParamMax=[]  KbOutMin=[]  KbOutMax=[]  KtOutMin=[]  KtOutMax=[]  IntegratorOutMin=[]  IntegratorOutMax=[]  FilterOutMin=[]  FilterOutMax=[]  SumI1OutMin=[]  SumI1OutMax=[]  SumI2OutMin=[]  SumI2OutMax=[]  SumI3OutMin=[]  SumI3OutMax=[]  SumI4OutMin=[]  SumI4OutMax=[]  SumDOutMin=[]  SumDOutMax=[]  DifferentiatorOutMin=[]  DifferentiatorOutMax=[]  FilterDiffOutCoefMin=[]  FilterDiffOutCoefMax=[]  ReciprocalOutMin=[]  ReciprocalOutMax=[]  SumDenOutMin=[]  SumDenOutMax=[]  SumNumOutMin=[]  SumNumOutMax=[]  DivideOutMin=[]  DivideOutMax=[]  UdiffTsProdOutMin=[]  UdiffTsProdOutMax=[]  NTsProdOutMin=[]  NTsProdOutMax=[]  UintegralTsProdOutMin=[]  UintegralTsProdOutMax=[]  UngainTsProdOutMin=[]  UngainTsProdOutMax=[]  IntegratorContinuousStateAttributes=''  IntegratorStateMustResolveToSignalObject=off  IntegratorRTWStateStorageClass=Auto  FilterContinuousStateAttributes=''  FilterStateMustResolveToSignalObject=off  FilterRTWStateStorageClass=Auto  ParallelPVariant=InternalParameters  IdealPVariant=Disabled  IVariant=InternalParameters  DVariant=Disabled  IntegratorVariant=Discrete  SatVariant=Enabled  AWVariant=DiscClampingParallel  PCopyVariant=Disabled  TRVariant=Disabled  FdbkBlocksVariant=Feedback  IdealPFdbkVariant=Passthrough  SatFdbkVariant=Passthrough  DerivativeFilterVariant=Disabled  NVariant=Disabled  NCopyVariant=Disabled_SignalSpec  FilterICVariant=Disabled  IntegratorICVariant=InternalICs  ExternalResetVariant=ExternalReset  TRSumVariant=Passthrough  SumFdbkVariant=Enabled  SumVariant=Sum_PI  TsampFilterVariant=InternalTs  TsampNgainVariant=Passthrough  TsampIntegralVariant=Passthrough  ExternalSaturationOutDataTypeStr=Inherit: Same as second input  aMode=0
  PID_yaw : slpidlib/PID Controller  Controller=P  Form=Parallel  TimeDomain=Discrete-time  UseExternalTs=off  SampleTime=SampleTime  IntegratorMethod=Backward Euler  FilterMethod=Forward Euler  ControllerParametersSource=internal  P=Kpy  I=Kiz  UseKiTs=off  D=Kdz  N=Nz  UseFilter=on  TunerSelectOption=Transfer Function Based (PID Tuner App)  InitialConditionSource=internal  InitialConditionForIntegrator=0  InitialConditionForFilter=0  DifferentiatorICPrevScaledInput=0  ExternalReset=none  TrackingMode=off  Kt=1  LimitOutput=on  SatLimitsSource=internal  UpperSaturationLimit=MAX_CONTROL_ANGLE_RATE_Y  LowerSaturationLimit=-MAX_CONTROL_ANGLE_RATE_Y  LinearizeAsGain=off  AntiWindupMode=clamping  Kb=1  POutMin=[]  POutMax=[]  IOutMin=[]  IOutMax=[]  DOutMin=[]  DOutMax=[]  NOutMin=[]  NOutMax=[]  SumOutMin=[]  SumOutMax=[]  SaturationOutMin=[]  SaturationOutMax=[]  PParamMin=[]  PParamMax=[]  IParamMin=[]  IParamMax=[]  DParamMin=[]  DParamMax=[]  NParamMin=[]  NParamMax=[]  KbParamMin=[]  KbParamMax=[]  KtParamMin=[]  KtParamMax=[]  KbOutMin=[]  KbOutMax=[]  KtOutMin=[]  KtOutMax=[]  IntegratorOutMin=[]  IntegratorOutMax=[]  FilterOutMin=[]  FilterOutMax=[]  SumI1OutMin=[]  SumI1OutMax=[]  SumI2OutMin=[]  SumI2OutMax=[]  SumI3OutMin=[]  SumI3OutMax=[]  SumI4OutMin=[]  SumI4OutMax=[]  SumDOutMin=[]  SumDOutMax=[]  DifferentiatorOutMin=[]  DifferentiatorOutMax=[]  FilterDiffOutCoefMin=[]  FilterDiffOutCoefMax=[]  ReciprocalOutMin=[]  ReciprocalOutMax=[]  SumDenOutMin=[]  SumDenOutMax=[]  SumNumOutMin=[]  SumNumOutMax=[]  DivideOutMin=[]  DivideOutMax=[]  UdiffTsProdOutMin=[]  UdiffTsProdOutMax=[]  NTsProdOutMin=[]  NTsProdOutMax=[]  UintegralTsProdOutMin=[]  UintegralTsProdOutMax=[]  UngainTsProdOutMin=[]  UngainTsProdOutMax=[]  IntegratorContinuousStateAttributes=''  IntegratorStateMustResolveToSignalObject=off  IntegratorRTWStateStorageClass=Auto  FilterContinuousStateAttributes=''  FilterStateMustResolveToSignalObject=off  FilterRTWStateStorageClass=Auto  ParallelPVariant=InternalParameters  IdealPVariant=Disabled  IVariant=Disabled  DVariant=Disabled  IntegratorVariant=Disabled  SatVariant=Enabled  AWVariant=Disabled  PCopyVariant=Disabled  TRVariant=Disabled  FdbkBlocksVariant=Forward  IdealPFdbkVariant=Disabled  SatFdbkVariant=Disabled  DerivativeFilterVariant=Disabled  NVariant=Disabled  NCopyVariant=Disabled_SignalSpec  FilterICVariant=Disabled  IntegratorICVariant=Disabled  ExternalResetVariant=Disabled  TRSumVariant=Passthrough  SumFdbkVariant=Disabled  SumVariant=Passthrough_P  TsampFilterVariant=InternalTs  TsampNgainVariant=Passthrough  TsampIntegralVariant=Disabled_SignalSpec  ExternalSaturationOutDataTypeStr=Inherit: Same as second input  aMode=0
  Sum{,1..5} (6 alike) : Sum  Inputs=|+-
  des_roll : Outport
  des_pitch : Outport  Port=2
  des_r : Outport  Port=3
  des_vz : Outport  Port=4
  log : Outport  Port=5
  wires:
  des_alt/1 -> [des_z], Sum2/1  "des_alt"
  yaw_angle/1 -> Sum3/2, MATLAB Function/2(psi)
  Altitude Signal conditioning/1(z) -> Sum2/2  "alt"
  PID_Altitude/1 -> des_vz/1  "vz_cmd"
  vx/1 -> Sum/2  "vx"
  vy/1 -> Sum5/2  "vy"
  Sum2/1 -> PID_Altitude/1
  z/1 -> Altitude Signal conditioning/1(z_In)
  x/1 -> Sum1/2  "x"
  MATLAB Function/2(theta) -> PID Controller/1
  MATLAB Function/1(phi) -> PID Controller3/1
  Sum1/1 -> PID Controller1/1
  des_x/1 -> [des_x], Sum1/1  "des_x"
  des_y/1 -> [des_y], Sum4/1  "des_y"
  PID Controller/1 -> des_pitch/1
  y/1 -> Sum4/2  "y"
  Sum4/1 -> PID Controller2/1
  Sum/1 -> Mux/1
  Sum5/1 -> Mux/2
  Mux/1 -> MATLAB Function/1(eaxy)
  PID Controller3/1 -> des_roll/1
  reset_sig/1 -> PID Controller3/2, PID Controller/2, PID_Altitude/2
  PID Controller2/1 -> [des_vy], Sum5/1
  PID Controller1/1 -> [des_vx], Sum/1
  des_yaw/1 -> [des_yaw], Sum3/1  "des_alt"
  Sum3/1 -> PID_yaw/1
  PID_yaw/1 -> des_r/1  "r_cmd"
  Mux5/1 -> log/1
  [des_x] -> Mux5/1
  [des_y] -> Mux5/2
  [des_z] -> Mux5/3
  [des_vx] -> Mux5/4
  [des_vy] -> Mux5/5
  [des_yaw] -> Gain15/1
  Gain15/1 -> Mux5/6  "des_Y"

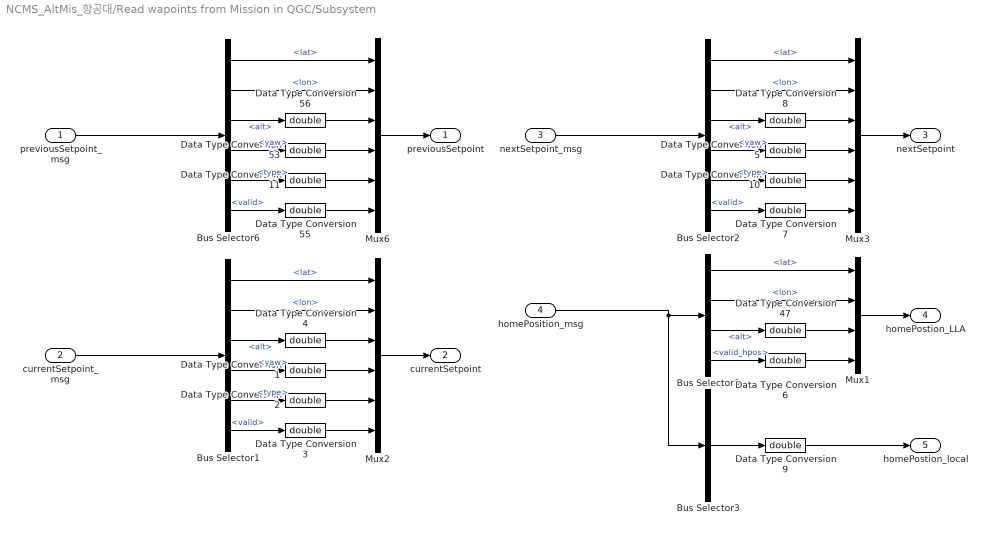
== system NCMS_AltMis_항공대/Read wapoints from Mission in QGC/Subsystem ==
  previousSetpoint_msg : Inport
  currentSetpoint_msg : Inport  Port=2
  nextSetpoint_msg : Inport  Port=3
  homePosition_msg : Inport  Port=4
  Bus Selector1 : BusSelector  OutputSignals=lat,lon,alt,yaw,type,valid
  Bus Selector2 : BusSelector  OutputSignals=lat,lon,alt,yaw,type,valid
  Bus Selector3 : BusSelector  OutputSignals=x,y,z,yaw  OutputAsBus=on
  Bus Selector6 : BusSelector  OutputSignals=lat,lon,alt,yaw,type,valid
  Bus Selector8 : BusSelector  OutputSignals=lat,lon,alt,valid_hpos
  Data Type Conversion{1..11,47,53,55..56} (15 alike) : DataTypeConversion  OutDataTypeStr=double  SaturateOnIntegerOverflow=off  RndMeth=Floor
  Mux1 : Mux
  Mux2 : Mux  Inputs=6
  Mux3 : Mux  Inputs=6
  Mux6 : Mux  Inputs=6
  previousSetpoint : Outport
  currentSetpoint : Outport  Port=2
  nextSetpoint : Outport  Port=3
  homePostion_LLA : Outport  Port=4
  homePostion_local : Outport  Port=5
  wires:
  previousSetpoint_msg/1 -> Bus Selector6/1
  Bus Selector8/1 -> Mux1/1  "<lat>"
  Bus Selector8/3 -> Data Type Conversion47/1  "<alt>"
  Bus Selector6/6 -> Data Type Conversion55/1  "<valid>"
  Bus Selector6/3 -> Data Type Conversion56/1  "<alt>"
  Bus Selector6/1 -> Mux6/1  "<lat>"
  Bus Selector6/4 -> Data Type Conversion53/1  "<yaw>"
  Data Type Conversion56/1 -> Mux6/3
  Bus Selector6/2 -> Mux6/2  "<lon>"
  Data Type Conversion53/1 -> Mux6/4
  Bus Selector8/2 -> Mux1/2  "<lon>"
  Mux1/1 -> homePostion_LLA/1
  Mux6/1 -> previousSetpoint/1
  Data Type Conversion3/1 -> Mux2/6
  Mux2/1 -> currentSetpoint/1
  Data Type Conversion1/1 -> Mux2/4
  Data Type Conversion4/1 -> Mux2/3
  currentSetpoint_msg/1 -> Bus Selector1/1
  Bus Selector1/2 -> Mux2/2  "<lon>"
  Data Type Conversion2/1 -> Mux2/5
  Bus Selector1/5 -> Data Type Conversion2/1  "<type>"
  Bus Selector1/4 -> Data Type Conversion1/1  "<yaw>"
  Bus Selector1/6 -> Data Type Conversion3/1  "<valid>"
  Bus Selector1/3 -> Data Type Conversion4/1  "<alt>"
  Bus Selector1/1 -> Mux2/1  "<lat>"
  Mux3/1 -> nextSetpoint/1
  Data Type Conversion5/1 -> Mux3/4
  Data Type Conversion8/1 -> Mux3/3
  nextSetpoint_msg/1 -> Bus Selector2/1
  Bus Selector2/2 -> Mux3/2  "<lon>"
  Bus Selector2/4 -> Data Type Conversion5/1  "<yaw>"
  Bus Selector2/6 -> Data Type Conversion7/1  "<valid>"
  Bus Selector2/3 -> Data Type Conversion8/1  "<alt>"
  Bus Selector2/1 -> Mux3/1  "<lat>"
  homePosition_msg/1 -> Bus Selector3/1, Bus Selector8/1
  Bus Selector3/1 -> Data Type Conversion9/1
  Data Type Conversion9/1 -> homePostion_local/1
  Bus Selector8/4 -> Data Type Conversion6/1  "<valid_hpos>"
  Data Type Conversion6/1 -> Mux1/4
  Data Type Conversion47/1 -> Mux1/3
  Bus Selector2/5 -> Data Type Conversion10/1  "<type>"
  Data Type Conversion10/1 -> Mux3/5
  Data Type Conversion7/1 -> Mux3/6
  Data Type Conversion55/1 -> Mux6/6
  Bus Selector6/5 -> Data Type Conversion11/1  "<type>"
  Data Type Conversion11/1 -> Mux6/5

== system NCMS_AltMis_항공대/Guidance/IDLE or Hovering/Maintain Current Yaw during IDLE ==
  yaw_In : Inport
  Constant : Constant  Value=0
  Delay : Delay  DelayLength=1  InitialCondition=1
  Enabled Subsystem2 : Subsystem  TreatAsAtomicUnit=on
  yaw_Out : Outport
  wires:
  Delay/1 -> Enabled Subsystem2/Enable
  Constant/1 -> Delay/1
  yaw_In/1 -> Enabled Subsystem2/1(yaw_In)
  Enabled Subsystem2/1(yaw_Out) -> yaw_Out/1

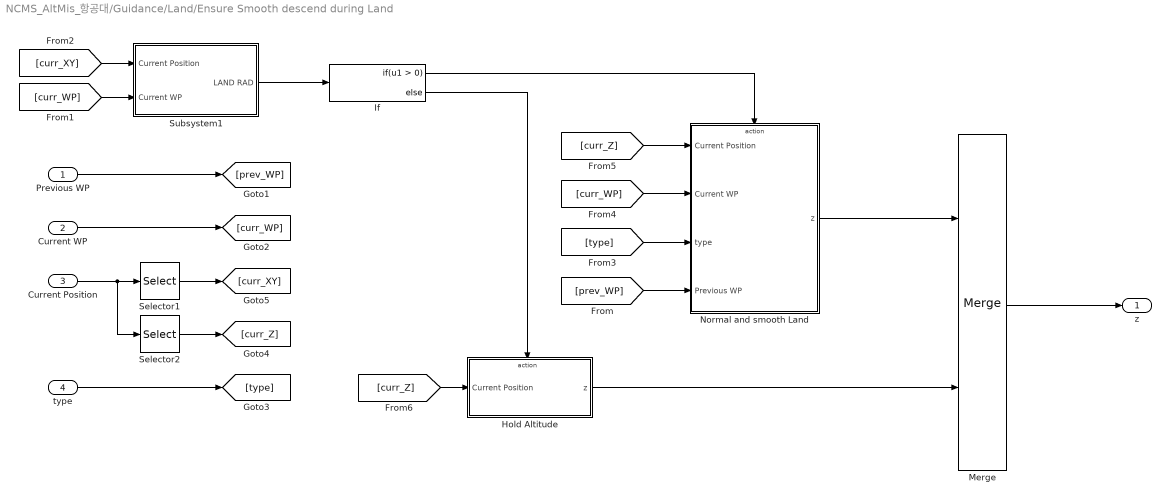
== system NCMS_AltMis_항공대/Guidance/Land/Ensure Smooth descend during Land ==
  Previous WP : Inport
  Current WP : Inport  Port=2
  Current Position : Inport  Port=3
  type : Inport  Port=4
  Hold Altitude : Subsystem  TreatAsAtomicUnit=on
  If : If
  Merge : Merge
  Normal and smooth Land : Subsystem  TreatAsAtomicUnit=on
  Selector1 : Selector  InputPortWidth=4  IndexOptions=Index vector (dialog)  Indices=[1 2]  OutputSizes=1
  Selector2 : Selector  InputPortWidth=4  IndexOptions=Index vector (dialog)  Indices=3  OutputSizes=1
  Subsystem1 : Subsystem
  z : Outport
  wires:
  Subsystem1/1(LAND RAD) -> If/1
  If/1 -> Normal and smooth Land/Action
  Merge/1 -> z/1
  Normal and smooth Land/1(z) -> Merge/1
  Current Position/1 -> Selector2/1, Selector1/1
  Previous WP/1 -> [prev_WP]
  Current WP/1 -> [curr_WP]
  type/1 -> [type]
  [curr_WP] -> Subsystem1/2(Current WP)
  [type] -> Normal and smooth Land/3(type)
  [prev_WP] -> Normal and smooth Land/4(Previous WP)
  [curr_WP] -> Normal and smooth Land/2(Current WP)
  If/2 -> Hold Altitude/Action
  Hold Altitude/1(z) -> Merge/2
  Selector2/1 -> [curr_Z]
  Selector1/1 -> [curr_XY]
  [curr_XY] -> Subsystem1/1(Current Position)
  [curr_Z] -> Normal and smooth Land/1(Current Position)
  [curr_Z] -> Hold Altitude/1(Current Position)

== system NCMS_AltMis_항공대/Guidance/Land/Maintain Current Yaw during Land ==
  yaw_In : Inport
  Constant : Constant  Value=0
  Delay : Delay  DelayLength=1  InitialCondition=1
  Enabled Subsystem2 : Subsystem  TreatAsAtomicUnit=on
  yaw_Out : Outport
  wires:
  Delay/1 -> Enabled Subsystem2/Enable
  Constant/1 -> Delay/1
  yaw_In/1 -> Enabled Subsystem2/1(yaw_In)
  Enabled Subsystem2/1(yaw_Out) -> yaw_Out/1

== system NCMS_AltMis_항공대/Guidance/Take-off/Ensure smooth ascend during Takeoff ==
  " " : Inport
  Delay : Delay  DelayLength=1
  Gain : Gain  Gain=-1
  Gain1 : Gain  Gain=-1
  Rate : Constant  Value=0.01
  Relational Operator : RelationalOperator  Operator=<=  OutDataTypeStr=boolean  RndMeth=Simplest  InputSameDT=off
  Sum : Sum  Inputs=|++
  Switch : Switch  Criteria=u2 > Threshold  SaturateOnIntegerOverflow=off  InputSameDT=off
  Out1 : Outport
  wires:
  Rate/1 -> Sum/1
  Gain/1 -> Out1/1
  Relational Operator/1 -> Switch/2
  Switch/1 -> Gain/1
  " "/1 -> Gain1/1
  Sum/1 -> Relational Operator/2, Switch/3, Delay/1
  Gain1/1 -> Switch/1, Relational Operator/1
  Delay/1 -> Sum/2

== system NCMS_AltMis_항공대/Guidance/Take-off/Maintain Current Yaw during TakeOff ==
  yaw_In : Inport
  Constant : Constant  Value=0
  Delay : Delay  DelayLength=1  InitialCondition=1
  Enabled Subsystem2 : Subsystem  TreatAsAtomicUnit=on
  yaw_Out : Outport
  wires:
  yaw_In/1 -> Enabled Subsystem2/1(yaw_In)
  Enabled Subsystem2/1(yaw_Out) -> yaw_Out/1
  Delay/1 -> Enabled Subsystem2/Enable
  Constant/1 -> Delay/1

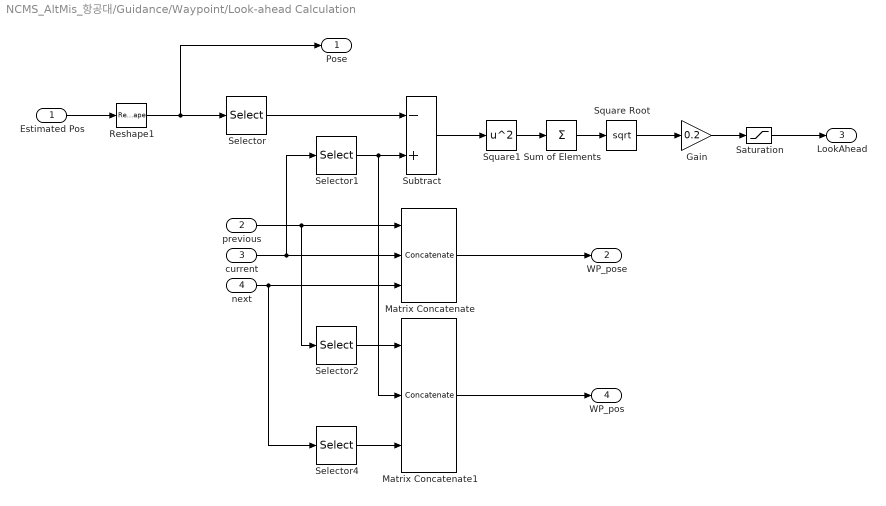
== system NCMS_AltMis_항공대/Guidance/Waypoint/Look-ahead Calculation ==
  Estimated Pos : Inport
  previous : Inport  Port=2
  current : Inport  Port=3
  next : Inport  Port=4
  Gain : Gain  Gain=0.2
  Matrix Concatenate : Concatenate  NumInputs=3  Mode=Multidimensional array
  Matrix Concatenate1 : Concatenate  NumInputs=3  Mode=Multidimensional array
  Reshape1 : Reshape
  Saturation : Saturate  UpperLimit=1.5  LowerLimit=0.5
  Selector{,1..2,4} (4 alike) : Selector  InputPortWidth=4  IndexOptions=Index vector (dialog)  Indices=[1 2 3]  OutputSizes=1
  Square Root : Sqrt
  Square1 : Math  Operator=square
  Subtract : Sum  Inputs=-+
  Sum of Elements : Sum  Inputs=+
  Pose : Outport
  WP_pose : Outport  Port=2
  LookAhead : Outport  Port=3
  WP_pos : Outport  Port=4
  wires:
  next/1 -> Selector4/1, Matrix Concatenate/3
  Matrix Concatenate/1 -> WP_pose/1
  previous/1 -> Selector2/1, Matrix Concatenate/1
  Gain/1 -> Saturation/1
  Estimated Pos/1 -> Reshape1/1
  Saturation/1 -> LookAhead/1
  Square Root/1 -> Gain/1
  Sum of Elements/1 -> Square Root/1
  Square1/1 -> Sum of Elements/1
  Subtract/1 -> Square1/1
  Reshape1/1 -> Pose/1, Selector/1
  current/1 -> Selector1/1, Matrix Concatenate/2
  Selector/1 -> Subtract/1
  Selector1/1 -> Matrix Concatenate1/2, Subtract/2
  Matrix Concatenate1/1 -> WP_pos/1
  Selector2/1 -> Matrix Concatenate1/1
  Selector4/1 -> Matrix Concatenate1/3

== system NCMS_AltMis_항공대/Guidance/Waypoint/Output signal conditioning ==
  Current Position : Inport
  LookAhead Point : Inport  Port=2
  Desired Yaw : Inport  Port=3
  Waypoint Type : Inport  Port=4
  Compare To Constant : simulink/Logic and Bit Operations/Compare To Constant  relop===  const=5  OutDataTypeStr=boolean
  Constant : Constant  Value=0  SampleTime=-1
  IsNaN : RelationalOperator  Operator=isNaN  OutDataTypeStr=boolean  RndMeth=Simplest  InputSameDT=off
  IsNaN1 : RelationalOperator  Operator=isNaN  OutDataTypeStr=boolean  RndMeth=Simplest  InputSameDT=off
  Matrix Concatenate1 : Concatenate  Mode=Multidimensional array  ConcatenateDimension=2
  OR : Logic  Operator=OR  IconShape=distinctive  AllPortsSameDT=off  OutDataTypeStr=boolean
  OR1 : Logic  Operator=OR  Inputs=1  IconShape=distinctive  AllPortsSameDT=off  OutDataTypeStr=boolean
  Reshape2 : Reshape  OutputDimensionality=Row vector (2-D)
  Reshape3 : Reshape  OutputDimensionality=Row vector (2-D)
  Switch : Switch  Criteria=u2 ~= 0  SaturateOnIntegerOverflow=off  InputSameDT=off
  Switch1 : Switch  Criteria=u2 > Threshold  SaturateOnIntegerOverflow=off  InputSameDT=off
  Transpose1 : Math  Operator=transpose
  xyzYaw : Outport
  wires:
  IsNaN1/1 -> OR1/1
  Reshape2/1 -> Matrix Concatenate1/2
  Matrix Concatenate1/1 -> Switch1/3
  OR/1 -> Switch1/2
  LookAhead Point/1 -> IsNaN1/1, Transpose1/1
  Compare To Constant/1 -> OR/2
  Transpose1/1 -> Matrix Concatenate1/1
  IsNaN/1 -> Switch/2
  Reshape3/1 -> Switch1/1
  Waypoint Type/1 -> Compare To Constant/1
  Switch1/1 -> xyzYaw/1
  Current Position/1 -> Reshape3/1
  OR1/1 -> OR/1
  Constant/1 -> Switch/1
  Switch/1 -> Reshape2/1
  Desired Yaw/1 -> Switch/3, IsNaN/1

== system NCMS_AltMis_항공대/Postion Controller/Position Controller/Altitude Signal conditioning ==
  z_In : Inport
  Constant : Constant  Value=0
  Saturation Dynamic : simulink/Discontinuities/Saturation Dynamic  OutMin=[]  OutMax=[]  OutDataTypeStr=Inherit: Same as second input  OutDataType=fixdt(1, 16)  OutScaling=2^-10  DoSatur=off
  z : Outport
  wires:
  z_In/1 -> Saturation Dynamic/3, Saturation Dynamic/2
  Saturation Dynamic/1 -> z/1  "alt"
  Constant/1 -> Saturation Dynamic/1

== system NCMS_AltMis_항공대/Guidance/IDLE or Hovering/Maintain Current Yaw during IDLE/Enabled Subsystem2 ==
  yaw_In : Inport
  Enable : EnablePort
  yaw_Out : Outport
  wires:
  yaw_In/1 -> yaw_Out/1

== system NCMS_AltMis_항공대/Guidance/Land/Ensure Smooth descend during Land/Hold Altitude ==
  Current Position : Inport
  Action Port : ActionPort  InitializeStates=reset  ActionPortLabel=else
  z : Outport
  wires:
  Current Position/1 -> z/1
